simulink model "test_pi_av_formation_event_gazebodirected23a"  (R2023a)
settings: Solver=FixedStepAuto  StartTime=0.0  StopTime=inf  RelTol=1e-3
undefined symbols (not defined in the file or in its folder): angular, DiscIntNeverNeededParam, linear
libraries: ros2lib x28, simulink x8, robotcorelib x8
(part 3 of 4)

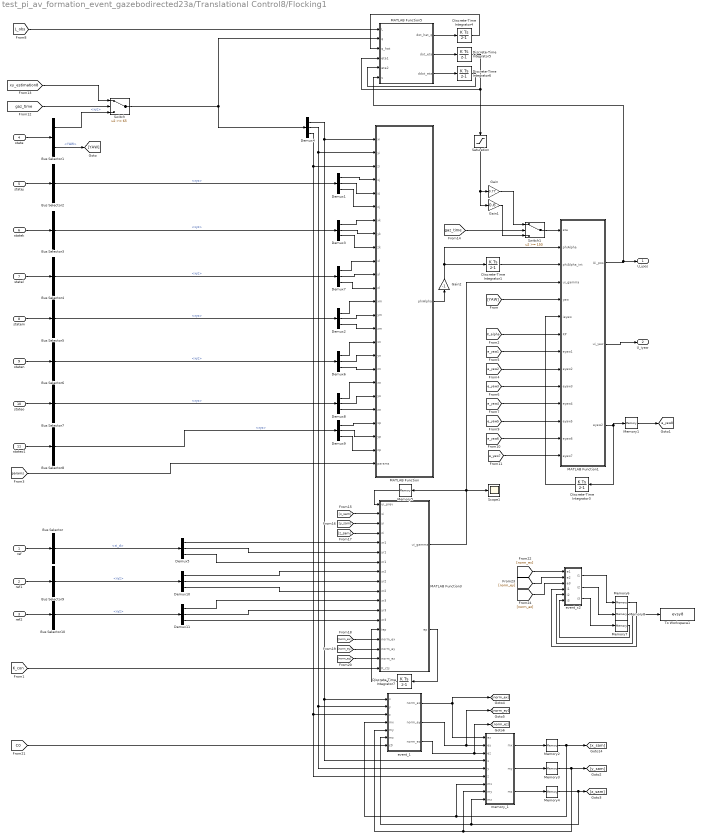
== system test_pi_av_formation_event_gazebodirected23a/Translational Control8/Flocking1 ==
  ref : Inport
  ref1 : Inport  Port=2
  ref2 : Inport  Port=3
  state : Inport  Port=4
  statej : Inport  Port=5
  statek : Inport  Port=6
  statel : Inport  Port=7
  statem : Inport  Port=8
  staten : Inport  Port=9
  stateo : Inport  Port=10
  stateo1 : Inport  Port=11
  Bus Selector : BusSelector  OutputSignals=xi_d
  Bus Selector1 : BusSelector  OutputSignals=xyz,YAW
  Bus Selector{2..10} (9 alike) : BusSelector  OutputSignals=xyz
  Demux{1..11} (11 alike) : Demux  Outputs=3
  Discrete-Time Integrator1 : DiscreteIntegrator  SampleTime=-1  LimitOutput=on  UpperSaturationLimit=2  LowerSaturationLimit=-2  ICPrevOutput=DiscIntNeverNeededParam  ICPrevScaledInput=DiscIntNeverNeededParam
  Discrete-Time Integrator3 : DiscreteIntegrator  SampleTime=-1  LimitOutput=on  UpperSaturationLimit=1  LowerSaturationLimit=-1  ICPrevOutput=DiscIntNeverNeededParam  ICPrevScaledInput=DiscIntNeverNeededParam
  Discrete-Time Integrator4 : DiscreteIntegrator  SampleTime=-1  LimitOutput=on  UpperSaturationLimit=5  LowerSaturationLimit=-5  ICPrevOutput=DiscIntNeverNeededParam  ICPrevScaledInput=DiscIntNeverNeededParam
  Discrete-Time Integrator5 : DiscreteIntegrator  SampleTime=-1  LimitOutput=on  UpperSaturationLimit=5  LowerSaturationLimit=-5  ICPrevOutput=DiscIntNeverNeededParam  ICPrevScaledInput=DiscIntNeverNeededParam
  Discrete-Time Integrator6 : DiscreteIntegrator  SampleTime=-1  LimitOutput=on  UpperSaturationLimit=0.4  LowerSaturationLimit=-0.4  ICPrevOutput=DiscIntNeverNeededParam  ICPrevScaledInput=DiscIntNeverNeededParam
  Discrete-Time Integrator7 : DiscreteIntegrator  SampleTime=-1  LimitOutput=on  UpperSaturationLimit=2  LowerSaturationLimit=-2  ICPrevOutput=DiscIntNeverNeededParam  ICPrevScaledInput=DiscIntNeverNeededParam
  Gain : Gain  Gain=0.77
  Gain1 : Gain  Gain=0.6
  Gain2 : Gain  Gain=-1
  MATLAB Function : MATLAB Function  TreatAsAtomicUnit=on
  MATLAB Function1 : MATLAB Function  TreatAsAtomicUnit=on
  MATLAB Function3 : MATLAB Function  TreatAsAtomicUnit=on
  MATLAB Function5 : MATLAB Function  TreatAsAtomicUnit=on
  Memory1 : Memory  InitialCondition=1
  Memory{2..4,6..8} (6 alike) : Memory
  Memory5 : Memory  InitialCondition=[0 0 0]'
  Saturation : Saturate  UpperLimit=1  LowerLimit=-1
  Scope1 : Scope
  Switch : Switch  Threshold=65  SaturateOnIntegerOverflow=off  InputSameDT=off
  Switch1 : Switch  Threshold=150  SaturateOnIntegerOverflow=off  InputSameDT=off
  To Workspace1 : ToWorkspace  VariableName=evsy8  SampleTime=-1
  event_1 : MATLAB Function  TreatAsAtomicUnit=on
  event_x2 : MATLAB Function  TreatAsAtomicUnit=on
  memory_1 : MATLAB Function  TreatAsAtomicUnit=on
  U_ipos : Outport  VectorParamsAs1DForOutWhenUnconnected=off
  U_iyaw : Outport  Port=2  VectorParamsAs1DForOutWhenUnconnected=off
  tag scope: e_yaw8=global
  wires:
  [e_yaw7] -> MATLAB Function1/14(eyaw7)
  Bus Selector8/1 -> Demux9/1  "<xyz>"
  Demux9/3 -> MATLAB Function/24(zp)
  Demux9/1 -> MATLAB Function/22(xp)
  Demux9/2 -> MATLAB Function/23(yp)
  stateo1/1 -> Bus Selector8/1
  ref/1 -> Bus Selector/1
  state/1 -> Bus Selector1/1
  Bus Selector/1 -> Demux5/1  "<xi_d>"
  statej/1 -> Bus Selector2/1
  Bus Selector2/1 -> Demux1/1  "<xyz>"
  Demux1/1 -> MATLAB Function/4(xj)
  Demux1/2 -> MATLAB Function/5(yj)
  Discrete-Time Integrator1/1 -> MATLAB Function1/3(phiAlpha_int)
  statek/1 -> Bus Selector3/1
  Demux3/1 -> MATLAB Function/7(xk)
  Demux3/2 -> MATLAB Function/8(yk)
  Bus Selector3/1 -> Demux3/1  "<xyz>"
  MATLAB Function/1(phiAlpha) -> Gain2/1
  Demux3/3 -> MATLAB Function/9(zk)
  Demux1/3 -> MATLAB Function/6(zj)
  statel/1 -> Bus Selector4/1
  Demux7/1 -> MATLAB Function/10(xl)
  Demux7/2 -> MATLAB Function/11(yl)
  Demux7/3 -> MATLAB Function/12(zl)
  Bus Selector4/1 -> Demux7/1  "<xyz>"
  Bus Selector1/2 -> [YAW]  "<YAW>"
  [YAW] -> MATLAB Function1/5(yaw)
  MATLAB Function1/2(ui_yaw) -> U_iyaw/1
  MATLAB Function1/3(eyaw2) -> Discrete-Time Integrator3/1, Memory1/1
  Discrete-Time Integrator3/1 -> MATLAB Function1/6(ieyaw)
  [K_alpha] -> MATLAB Function1/7(KP)
  [params] -> MATLAB Function/25(params)
  statem/1 -> Bus Selector5/1
  Bus Selector5/1 -> Demux2/1  "<xyz>"
  Demux2/1 -> MATLAB Function/13(xm)
  Demux2/2 -> MATLAB Function/14(ym)
  Demux2/3 -> MATLAB Function/15(zm)
  Memory1/1 -> [e_yaw8]
  [e_yaw1] -> MATLAB Function1/8(eyaw1)
  [e_yaw3] -> MATLAB Function1/10(eyaw3)
  [e_yaw4] -> MATLAB Function1/11(eyaw4)
  [e_yaw2] -> MATLAB Function1/9("eyaw2 ")
  Discrete-Time Integrator4/1 -> MATLAB Function5/3(q_hat)
  Discrete-Time Integrator5/1 -> Saturation/1, MATLAB Function5/4(eta1)
  [L_obs] -> MATLAB Function5/1(L)
  MATLAB Function5/1(dot_hat_q) -> Discrete-Time Integrator4/1
  MATLAB Function1/1(Ui_pos) -> MATLAB Function5/6(u), U_ipos/1
  MATLAB Function5/2(dot_eta) -> Discrete-Time Integrator5/1
  Discrete-Time Integrator6/1 -> MATLAB Function5/5(eta2)
  MATLAB Function5/3(ddot_eta) -> Discrete-Time Integrator6/1
  staten/1 -> Bus Selector6/1
  Demux6/1 -> MATLAB Function/16(xn)
  Demux6/2 -> MATLAB Function/17(yn)
  Demux6/3 -> MATLAB Function/18(zn)
  Bus Selector6/1 -> Demux6/1  "<xyz>"
  [e_yaw5] -> MATLAB Function1/12(eyaw5)
  stateo/1 -> Bus Selector7/1
  Demux8/1 -> MATLAB Function/19(xo)
  Demux8/2 -> MATLAB Function/20(yo)
  Demux8/3 -> MATLAB Function/21(zo)
  Bus Selector7/1 -> Demux8/1  "<xyz>"
  [e_yaw6] -> MATLAB Function1/13(eyaw6)
  [xy_estimation8] -> Switch/1
  [gaz_time] -> Switch/2
  Bus Selector1/1 -> Switch/3  "<xyz>"
  Switch/1 -> MATLAB Function5/2(q), Demux4/1
  Bus Selector9/1 -> Demux10/1  "<xyz>"
  ref1/1 -> Bus Selector9/1
  ref2/1 -> Bus Selector10/1
  Bus Selector10/1 -> Demux11/1  "<xyz>"
  Saturation/1 -> Gain1/1, Gain/1
  Switch1/1 -> MATLAB Function1/1(eta)
  Gain1/1 -> Switch1/3
  Gain/1 -> Switch1/1
  [gaz_time] -> Switch1/2
  event_1/3(norm_ez) -> [norm_ez], memory_1/3(ez)
  Memory2/1 -> memory_1/7("mx "), event_1/4(mx), [x_sam]
  [norm_ez] -> MATLAB Function3/17(norm_ez)
  MATLAB Function3/1(ui_gamma) -> MATLAB Function1/4(ui_gamma), Scope1/1, Memory5/1
  Memory5/1 -> MATLAB Function3/1(ui_prev)
  memory_1/1(mx) -> Memory2/1
  Memory3/1 -> [y_sam], memory_1/8("my "), event_1/5(my)
  event_1/1(norm_ex) -> [norm_ex], memory_1/1(ex)
  memory_1/3(mz) -> Memory4/1
  MATLAB Function3/2(ep) -> Discrete-Time Integrator7/1
  [norm_ey] -> MATLAB Function3/16(norm_ey)
  [norm_ex] -> MATLAB Function3/15(norm_ex)
  memory_1/2(my) -> Memory3/1
  [x_sam] -> MATLAB Function3/2(xi)
  Discrete-Time Integrator7/1 -> MATLAB Function3/14(iep)
  event_1/2(norm_ey) -> [norm_ey], memory_1/2(ey)
  [y_sam] -> MATLAB Function3/3(yi)
  [z_sam] -> MATLAB Function3/4(zi)
  Demux4/1 -> memory_1/4(x), event_1/1(x), MATLAB Function/1(xi)
  Memory4/1 -> memory_1/9("mz "), event_1/6(mz), [z_sam]
  Demux4/2 -> memory_1/5(y), event_1/2(y), MATLAB Function/2(yi)
  Demux4/3 -> memory_1/6(z), event_1/3(z), MATLAB Function/3(zi)
  Demux11/1 -> MATLAB Function3/11(xr3)
  Demux10/1 -> MATLAB Function3/8(xr2)
  Demux11/2 -> MATLAB Function3/12(yr3)
  Demux5/1 -> MATLAB Function3/5(xr1)
  Demux10/2 -> MATLAB Function3/9(yr2)
  Demux11/3 -> MATLAB Function3/13(zr3)
  Demux5/2 -> MATLAB Function3/6(yr1)
  Demux10/3 -> MATLAB Function3/10(zr2)
  Demux5/3 -> MATLAB Function3/7(zr1)
  [K_con] -> MATLAB Function3/18(K_cts)
  [C0] -> event_1/7(c0)
  Gain2/1 -> MATLAB Function1/2(phiAlpha), Discrete-Time Integrator1/1
  Memory7/1 -> event_x2/6("i3 ")
  [norm_ez] -> event_x2/3(e3)
  [norm_ex] -> event_x2/1(e1)
  event_x2/2(i2) -> Memory8/1
  Memory8/1 -> To Workspace1/1, event_x2/5("i2 ")
  event_x2/1(i1) -> Memory6/1
  Memory6/1 -> event_x2/4("i1 ")
  event_x2/3(i3) -> Memory7/1
  [norm_ey] -> event_x2/2(e2)

== matlab function test_pi_av_formation_event_gazebodirected23a/Translational Control3/Flocking1/event_1 ==
  data: x input; y input; z input; mx input; my input; mz input; norm_ex output; norm_ey output; c0 input; norm_ez output
function [norm_ex, norm_ey, norm_ez] = fcn(x, y, z, mx, my, mz, c0)

cx = c0(1); cy = c0(2); cz = c0(3); 

norm_ex = abs((mx-x)) - cx;
norm_ey = abs((my-y)) - cy;
norm_ez = abs((mz-z)) - cz;

== matlab function test_pi_av_formation_event_gazebodirected23a/Translational Control3/Flocking1/memory_1 ==
  data: ex input; ey input; mx output; ez input; x input; y input; z input; mx input; my input; mz input; my output; mz output
function [mx, my, mz] = fcn(ex, ey, ez, x, y, z, mx, my, mz)

if ex >= 0
    mx = x;    
else
    mx = mx;
end

if ey >= 0
    my = y;    
else
    my = my;
end

if ez >= 0
    mz = z;    
else
    mz = mz;
end

== matlab function test_pi_av_formation_event_gazebodirected23a/Translational Control4/Flocking1/event_1 ==
  data: x input; y input; z input; mx input; my input; mz input; norm_ex output; norm_ey output; c0 input; norm_ez output
function [norm_ex, norm_ey, norm_ez] = fcn(x, y, z, mx, my, mz, c0)

cx = c0(1); cy = c0(2); cz = c0(3); 

norm_ex = abs((mx-x)) - cx;
norm_ey = abs((my-y)) - cy;
norm_ez = abs((mz-z)) - cz;

== matlab function test_pi_av_formation_event_gazebodirected23a/Translational Control4/Flocking1/memory_1 ==
  data: ex input; ey input; mx output; ez input; x input; y input; z input; mx input; my input; mz input; my output; mz output
function [mx, my, mz] = fcn(ex, ey, ez, x, y, z, mx, my, mz)

if ex >= 0
    mx = x;    
else
    mx = mx;
end

if ey >= 0
    my = y;    
else
    my = my;
end

if ez >= 0
    mz = z;    
else
    mz = mz;
end

== matlab function test_pi_av_formation_event_gazebodirected23a/MATLAB Function1 ==
  data: sec input; gaz_time output; nanosec input
function gaz_time = fcn(sec, nanosec)

nanosec1 = double(nanosec)/1000000000; %*10^(-9);

sec1 = double(sec);

gaz_time = sec1 + nanosec1;

== matlab function test_pi_av_formation_event_gazebodirected23a/Translational Control5/Flocking1/event_1 ==
  data: x input; y input; z input; mx input; my input; mz input; norm_ex output; norm_ey output; c0 input; norm_ez output
function [norm_ex, norm_ey, norm_ez] = fcn(x, y, z, mx, my, mz, c0)

cx = c0(1); cy = c0(2); cz = c0(3); 

norm_ex = abs((mx-x)) - cx;
norm_ey = abs((my-y)) - cy;
norm_ez = abs((mz-z)) - cz;

== matlab function test_pi_av_formation_event_gazebodirected23a/Translational Control5/Flocking1/memory_1 ==
  data: ex input; ey input; mx output; ez input; x input; y input; z input; mx input; my input; mz input; my output; mz output
function [mx, my, mz] = fcn(ex, ey, ez, x, y, z, mx, my, mz)

if ex >= 0
    mx = x;    
else
    mx = mx;
end

if ey >= 0
    my = y;    
else
    my = my;
end

if ez >= 0
    mz = z;    
else
    mz = mz;
end

== matlab function test_pi_av_formation_event_gazebodirected23a/Translational Control6/Flocking1/event_1 ==
  data: x input; y input; z input; mx input; my input; mz input; norm_ex output; norm_ey output; c0 input; norm_ez output
function [norm_ex, norm_ey, norm_ez] = fcn(x, y, z, mx, my, mz, c0)

cx = c0(1); cy = c0(2); cz = c0(3); 

norm_ex = abs((mx-x)) - cx;
norm_ey = abs((my-y)) - cy;
norm_ez = abs((mz-z)) - cz;

== matlab function test_pi_av_formation_event_gazebodirected23a/Translational Control6/Flocking1/memory_1 ==
  data: ex input; ey input; mx output; ez input; x input; y input; z input; mx input; my input; mz input; my output; mz output
function [mx, my, mz] = fcn(ex, ey, ez, x, y, z, mx, my, mz)

if ex >= 0
    mx = x;    
else
    mx = mx;
end

if ey >= 0
    my = y;    
else
    my = my;
end

if ez >= 0
    mz = z;    
else
    mz = mz;
end

== matlab function test_pi_av_formation_event_gazebodirected23a/Subsystem/dist_AVT ==
  data: meas input; u_B input; dU output; dAVT output; avt_pars input
function [dU,dAVT]  = fcn(meas, u_B, avt_pars)

%Vector separation
d1 = meas(1);
d2 = meas(2);
d3 = meas(3);
d4 = meas(4);
d5 = meas(5);
d6 = meas(6);
d7 = meas(7);

avtpars = avt_pars(1:4);
inc = avtpars(1);
dec = avtpars(2);
min = avtpars(3);
max = avtpars(4);

%% memory variables
d_avt1 = u_B(1);
adjustment1 = u_B(2);
s_adjust1 = u_B(3);

d_avt2 = u_B(4);
adjustment2 = u_B(5);
s_adjust2 = u_B(6);

d_avt3 = u_B(7);
adjustment3 = u_B(8);
s_adjust3 = u_B(9);

d_avt4 = u_B(10);
adjustment4 = u_B(11);
s_adjust4 = u_B(12);

d_avt5 = u_B(13);
adjustment5 = u_B(14);
s_adjust5 = u_B(15);

d_avt6 = u_B(16);
adjustment6 = u_B(17);
s_adjust6 = u_B(18);

d_avt7 = u_B(19);
adjustment7 = u_B(20);
s_adjust7 = u_B(21);

%%
du1 = AVTfun(d_avt1, d1, adjustment1, s_adjust1, min, max, inc, dec);

du2 = AVTfun(d_avt2, d2, adjustment2, s_adjust2, min, max, inc, dec);

du3 = AVTfun(d_avt3, d3, adjustment3, s_adjust3, min, max, inc, dec);

du4 = AVTfun(d_avt4, d4, adjustment4, s_adjust4, min, max, inc, dec);

du5 = AVTfun(d_avt5, d5, adjustment5, s_adjust5, min, max, inc, dec);

du6 = AVTfun(d_avt6, d6, adjustment6, s_adjust6, min, max, inc, dec);

du7 = AVTfun(d_avt7, d7, adjustment7, s_adjust7, min, max, inc, dec);

dU = [du1;du2;du3;du4;du5;du6;du7];
dAVT = [du1(1);du2(1);du3(1);du4(1);du5(1);du6(1);du7(1)];

== matlab function test_pi_av_formation_event_gazebodirected23a/MATLAB Function ==
  data: data input; y output
function y = fcn(data)

DATA = data(1:20);
d1 = awgn(double(DATA(1)), 33, 'measured');
d2 = awgn(double(DATA(2)), 33, 'measured');
d3 = awgn(double(DATA(3)), 33, 'measured');
d4 = awgn(double(DATA(4)), 33, 'measured');
d5 = awgn(double(DATA(5)), 33, 'measured');
d6 = awgn(double(DATA(6)), 33, 'measured');
d7 = awgn(double(DATA(7)), 33, 'measured');
y = [d1;d2;d3;d4;d5;d6;d7];

== matlab function test_pi_av_formation_event_gazebodirected23a/Subsystem/MATLAB Function6 ==
  data: X1 input; X2 input; X3 input; X4 input; X5 input; X6 input; X7 input; d_meas input; xyz output
function xyz = fcn(X1, X2, X3, X4, X5, X6, X7, d_meas)

%% Extract data from vectors
states1 = X1(1:3);
x1 = states1(1);
y1 = states1(2);
z1 = states1(3);

states2 = X2(1:3);
x2 = states2(1);
y2 = states2(2);
z2 = states2(3);

states3 = X3(1:3);
x3 = states3(1);
y3 = states3(2);
z3 = states3(3);

states4 = X4(1:3);
x4 = states4(1);
y4 = states4(2);
z4 = states4(3);

states5 = X5(1:3);
x5 = states5(1);
y5 = states5(2);
z5 = states5(3);

states6 = X6(1:3);
x6 = states6(1);
y6 = states6(2);
z6 = states6(3);

states7 = X7(1:3);
x7 = states7(1);
y7 = states7(2);
z7 = states7(3);

r1 = d_meas(1);
r2 = d_meas(2);
r3 = d_meas(3);
r4 = d_meas(4);
r5 = d_meas(5);
r6 = d_meas(6);
r7 = d_meas(7);

xyz = multi_fun2(x1, y1, z1, r1, x2, y2, z2, r2, x3, y3, z3, r3, x4, y4, z4, r4, x5, y5, z5, r5, x6, y6, z6, r6, x7, y7, z7, r7);

== matlab function test_pi_av_formation_event_gazebodirected23a/Translational Control7/Flocking1/event_1 ==
  data: x input; y input; z input; mx input; my input; mz input; norm_ex output; norm_ey output; c0 input; norm_ez output
function [norm_ex, norm_ey, norm_ez] = fcn(x, y, z, mx, my, mz, c0)

cx = c0(1); cy = c0(2); cz = c0(3); 

norm_ex = abs((mx-x)) - cx;
norm_ey = abs((my-y)) - cy;
norm_ez = abs((mz-z)) - cz;

== matlab function test_pi_av_formation_event_gazebodirected23a/Translational Control7/Flocking1/memory_1 ==
  data: ex input; ey input; mx output; ez input; x input; y input; z input; mx input; my input; mz input; my output; mz output
function [mx, my, mz] = fcn(ex, ey, ez, x, y, z, mx, my, mz)

if ex >= 0
    mx = x;    
else
    mx = mx;
end

if ey >= 0
    my = y;    
else
    my = my;
end

if ez >= 0
    mz = z;    
else
    mz = mz;
end

== matlab function test_pi_av_formation_event_gazebodirected23a/Translational Control8/Flocking1/event_1 ==
  data: x input; y input; z input; mx input; my input; mz input; norm_ex output; norm_ey output; c0 input; norm_ez output
function [norm_ex, norm_ey, norm_ez] = fcn(x, y, z, mx, my, mz, c0)

cx = c0(1); cy = c0(2); cz = c0(3); 

norm_ex = abs((mx-x)) - cx;
norm_ey = abs((my-y)) - cy;
norm_ez = abs((mz-z)) - cz;

== matlab function test_pi_av_formation_event_gazebodirected23a/Translational Control8/Flocking1/memory_1 ==
  data: ex input; ey input; mx output; ez input; x input; y input; z input; mx input; my input; mz input; my output; mz output
function [mx, my, mz] = fcn(ex, ey, ez, x, y, z, mx, my, mz)

if ex >= 0
    mx = x;    
else
    mx = mx;
end

if ey >= 0
    my = y;    
else
    my = my;
end

if ez >= 0
    mz = z;    
else
    mz = mz;
end

== matlab function test_pi_av_formation_event_gazebodirected23a/Virtual_leader ==
  data: t input; xi_d output; dxi_d output; Xd input
function [xi_d, dxi_d]  = fcn(t, Xd)
%#codegen

f = 1/110;
radius=2;   %radius in meters

sel=1;      %inputs or parameters dont work! only local vars ...

if sel == 1
    if t < 90
       xd     =  0.5;
       xdotd  =  0;
           
       yd     = 0.5;
       ydotd  = 0;
           
       zd     = 1.3;  
       zdotd  = 0; 
           
       xi_d =[xd; yd; zd];
       dxi_d=[xdotd; ydotd; zdotd]; 
       
    elseif t < 120
        xd     =  0.4;
        xdotd  =  0;
            
        yd     = -0.4;
        ydotd  = 0;
            
        zd     = 2.5;  
        zdotd  = 0; 
            
        xi_d =[xd; yd; zd];
        dxi_d=[xdotd; ydotd; zdotd]; 
        
    elseif t < 220
       xd     = radius*sin(2*pi*f*t);
       xdotd  = radius*2*pi*f*cos(2*pi*f*t);
            
       yd     = radius*cos(2*pi*f*t);
       ydotd  = -radius*2*pi*f*sin(2*pi*f*t);
            
       zd     = 3;  %radius*cos(2*pi*f*t) + 5;
       zdotd  = 0;  %-radius*2*pi*f*sin(2*pi*f*t);
           
       xi_d =[xd; yd; zd];
       dxi_d=[xdotd; ydotd; zdotd];
    else
        xd     =  1;
        xdotd  =  0;
            
        yd     = 1;
        ydotd  = 0;
            
        zd     = 2;  
        zdotd  = 0; 
            
        xi_d =[xd; yd; zd];
        dxi_d=[xdotd; ydotd; zdotd];        
    end
end

 if(sel==2)
     xd     =  Xd(1);
     xdotd  =  0;
          
     yd     = Xd(2);
     ydotd  = 0;
          
     zd     = Xd(3);  
     zdotd  = 0; 
          
     xi_d =[xd; yd; zd];
     dxi_d=[xdotd; ydotd; zdotd]; 
     
 end

== matlab function test_pi_av_formation_event_gazebodirected23a/Translational Control2/Flocking1/event_x2 ==
  data: e1 input; e2 input; e3 input; i1 output; i1 input; i2 input; i3 input; i2 output; i3 output
function [i1, i2, i3]  = fcn(e1, e2, e3, i1, i2, i3)

if e1 >= 0
    e_1 = 1;
    i1 = i1+1;
else 
    e_1 = 0;
    i1 = i1;
end

if e2 >= 0
    e_2 = 1;
    i2 = i2 + 1;
else 
    e_2 = 0;
    i2 = i2;
end

if e3 >= 0
    e_3 = 1;
    i3 = i3 + 1;
else 
    e_3 = 0;
    i3 = i3;
end

== matlab function test_pi_av_formation_event_gazebodirected23a/Translational Control3/Flocking1/event_x2 ==
  data: e1 input; e2 input; e3 input; i1 output; i1 input; i2 input; i3 input; i2 output; i3 output
function [i1, i2, i3]  = fcn(e1, e2, e3, i1, i2, i3)

if e1 >= 0
    e_1 = 1;
    i1 = i1+1;
else 
    e_1 = 0;
    i1 = i1;
end

if e2 >= 0
    e_2 = 1;
    i2 = i2 + 1;
else 
    e_2 = 0;
    i2 = i2;
end

if e3 >= 0
    e_3 = 1;
    i3 = i3 + 1;
else 
    e_3 = 0;
    i3 = i3;
end

== matlab function test_pi_av_formation_event_gazebodirected23a/Translational Control4/Flocking1/event_x2 ==
  data: e1 input; e2 input; e3 input; i1 output; i1 input; i2 input; i3 input; i2 output; i3 output
function [i1, i2, i3]  = fcn(e1, e2, e3, i1, i2, i3)

if e1 >= 0
    e_1 = 1;
    i1 = i1+1;
else 
    e_1 = 0;
    i1 = i1;
end

if e2 >= 0
    e_2 = 1;
    i2 = i2 + 1;
else 
    e_2 = 0;
    i2 = i2;
end

if e3 >= 0
    e_3 = 1;
    i3 = i3 + 1;
else 
    e_3 = 0;
    i3 = i3;
end

== matlab function test_pi_av_formation_event_gazebodirected23a/Translational Control5/Flocking1/event_x2 ==
  data: e1 input; e2 input; e3 input; i1 output; i1 input; i2 input; i3 input; i2 output; i3 output
function [i1, i2, i3]  = fcn(e1, e2, e3, i1, i2, i3)

if e1 >= 0
    e_1 = 1;
    i1 = i1+1;
else 
    e_1 = 0;
    i1 = i1;
end

if e2 >= 0
    e_2 = 1;
    i2 = i2 + 1;
else 
    e_2 = 0;
    i2 = i2;
end

if e3 >= 0
    e_3 = 1;
    i3 = i3 + 1;
else 
    e_3 = 0;
    i3 = i3;
end

== matlab function test_pi_av_formation_event_gazebodirected23a/Translational Control6/Flocking1/event_x2 ==
  data: e1 input; e2 input; e3 input; i1 output; i1 input; i2 input; i3 input; i2 output; i3 output
function [i1, i2, i3]  = fcn(e1, e2, e3, i1, i2, i3)

if e1 >= 0
    e_1 = 1;
    i1 = i1+1;
else 
    e_1 = 0;
    i1 = i1;
end

if e2 >= 0
    e_2 = 1;
    i2 = i2 + 1;
else 
    e_2 = 0;
    i2 = i2;
end

if e3 >= 0
    e_3 = 1;
    i3 = i3 + 1;
else 
    e_3 = 0;
    i3 = i3;
end

== matlab function test_pi_av_formation_event_gazebodirected23a/Translational Control7/Flocking1/event_x2 ==
  data: e1 input; e2 input; e3 input; i1 output; i1 input; i2 input; i3 input; i2 output; i3 output
function [i1, i2, i3]  = fcn(e1, e2, e3, i1, i2, i3)

if e1 >= 0
    e_1 = 1;
    i1 = i1+1;
else 
    e_1 = 0;
    i1 = i1;
end

if e2 >= 0
    e_2 = 1;
    i2 = i2 + 1;
else 
    e_2 = 0;
    i2 = i2;
end

if e3 >= 0
    e_3 = 1;
    i3 = i3 + 1;
else 
    e_3 = 0;
    i3 = i3;
end

== matlab function test_pi_av_formation_event_gazebodirected23a/Translational Control2/Flocking1/MATLAB Function ==
  data: xi input; yi input; zi input; phiAlpha output; xj input; yj input; zj input; xk input; yk input; zk input; xl input; yl input; zl input; xm input; ym input; zm input; xn input; yn input; zn input; xo input; yo input; zo input; xp input; yp input; zp input; params input

function phiAlpha  = phiAlphaFcn(xi, yi, zi, xj, yj, zj, xk, yk, zk, xl, yl, zl, xm, ym, zm, xn, yn, zn, xo, yo, zo, xp, yp, zp, params)
    
    % Flocking parameters
    epsilon = params(1); a = params(2); b = params(3); c = params(4); d = params(5); h = params(6);

    e = abs(a - b) / sqrt(4*a*b) ;

    cAlpha = sigmaNormFun(c, epsilon) ;
    dAlpha = sigmaNormFun(d, epsilon) ;

    %%
    Pi = [xi;yi;zi] ;

    Pj = [xj;yj;zj] ;
    Pk = [xk;yk;zk] ;
    Pl = [xl;yl;zl] ;
    Pm = [xm;ym;zm] ;
    Pn = [xn;yn;zn] ;
    Po = [xo;yo;zo] ;
    Pp = [xp;yp;zp] ;

    %%
    sigmaNormj = sigmaNormFun(Pj - Pi, epsilon) ;
    nij = gradSigmaFun(Pj - Pi, epsilon) ;
    
    sigmaNormk = sigmaNormFun(Pk - Pi, epsilon) ;
    nik = gradSigmaFun(Pk - Pi, epsilon) ;

    sigmaNorml = sigmaNormFun(Pl - Pi, epsilon) ;
    nil = gradSigmaFun(Pl - Pi, epsilon) ;

    sigmaNormm = sigmaNormFun(Pm - Pi, epsilon) ;
    nim = gradSigmaFun(Pm - Pi, epsilon) ;

    sigmaNormn = sigmaNormFun(Pn - Pi, epsilon) ;
    nin = gradSigmaFun(Pn - Pi, epsilon) ;

    sigmaNormo = sigmaNormFun(Po - Pi, epsilon) ;
    nio = gradSigmaFun(Po - Pi, epsilon) ;

    sigmaNormp = sigmaNormFun(Pp - Pi, epsilon) ;
    nip = gradSigmaFun(Pp - Pi, epsilon) ;

    %%
    sigma1j = sigma1Fun(sigmaNormj - dAlpha + e) ;
    sigma1k = sigma1Fun(sigmaNormk - dAlpha + e) ;
    sigma1l = sigma1Fun(sigmaNorml - dAlpha + e) ;
    sigma1m = sigma1Fun(sigmaNormm - dAlpha + e) ;
    sigma1n = sigma1Fun(sigmaNormn - dAlpha + e) ;
    sigma1o = sigma1Fun(sigmaNormo - dAlpha + e) ;
    sigma1p = sigma1Fun(sigmaNormp - dAlpha + e) ;
            
    %% Position
    phiAlphaj = 0.5 * bumpFcn(sigmaNormj/cAlpha,h) * ((a+b)*sigma1j + (a-b)) ;
    phiAlphanij = phiAlphaj.* nij ;
    
    phiAlphak = 0.5 * bumpFcn(sigmaNormk/cAlpha,h) * ((a+b)*sigma1k + (a-b)) ;
    phiAlphanik = phiAlphak.* nik ;

    phiAlphal = 0.5 * bumpFcn(sigmaNorml/cAlpha,h) * ((a+b)*sigma1l + (a-b)) ;
    phiAlphanil = phiAlphal.* nil ;

    phiAlpham = 0.5 * bumpFcn(sigmaNormm/cAlpha,h) * ((a+b)*sigma1m + (a-b)) ;
    phiAlphanim = phiAlpham.* nim ;

    phiAlphan = 0.5 * bumpFcn(sigmaNormn/cAlpha,h) * ((a+b)*sigma1n + (a-b)) ;
    phiAlphanin = phiAlphan.* nin ;

    phiAlphao = 0.5 * bumpFcn(sigmaNormo/cAlpha,h) * ((a+b)*sigma1o + (a-b)) ;
    phiAlphanio = phiAlphao.* nio ;

    phiAlphap = 0.5 * bumpFcn(sigmaNormp/cAlpha,h) * ((a+b)*sigma1p + (a-b)) ;
    phiAlphanip = phiAlphap.* nip ;


    phiAlpha = phiAlphanij + phiAlphanik + phiAlphanil + phiAlphanim + phiAlphanin + phiAlphanio + phiAlphanip;

    
end

== matlab function test_pi_av_formation_event_gazebodirected23a/Translational Control8/Flocking1/event_x2 ==
  data: e1 input; e2 input; e3 input; i1 output; i1 input; i2 input; i3 input; i2 output; i3 output
function [i1, i2, i3]  = fcn(e1, e2, e3, i1, i2, i3)

if e1 >= 0
    e_1 = 1;
    i1 = i1+1;
else 
    e_1 = 0;
    i1 = i1;
end

if e2 >= 0
    e_2 = 1;
    i2 = i2 + 1;
else 
    e_2 = 0;
    i2 = i2;
end

if e3 >= 0
    e_3 = 1;
    i3 = i3 + 1;
else 
    e_3 = 0;
    i3 = i3;
end

== matlab function test_pi_av_formation_event_gazebodirected23a/continuous ==
  data: i output; t input; tp input; tp output; i input
function [i,tp] = fcn(t,tp,i)


%u = 0.1*cos(1.5*t) + 0.05*sin(t);         % x-component of vector field
%v = 0.1*sin(3*t) - 0.06*sin(0.5*t);      % y-component of vector field
if t > tp
    i = i + 1;
else 
    i = i;
end

== matlab function test_pi_av_formation_event_gazebodirected23a/Translational Control2/Flocking1/MATLAB Function1 ==
  data: eta input; phiAlpha input; phiAlpha_int input; ui_gamma input; yaw input; ieyaw input; Ui_pos output size=3; ui_yaw output; KP input; eyaw output size=1; eyaw1 input; eyaw3 input; eyaw4 input; eyaw5 input; eyaw6 input; eyaw7 input; eyaw8 input

function [Ui_pos, ui_yaw, eyaw]  = ctrlLaw(eta, phiAlpha, phiAlpha_int, ui_gamma, yaw, ieyaw, KP, eyaw1, eyaw3, eyaw4, eyaw5, eyaw6, eyaw7, eyaw8)  %, phiBetak, bikobs, phiBetanei, bikve
    
    % Control gains and parameters
    Kx = KP(1); Ky = KP(2); Kz = KP(3);
    Kix = KP(4); Kiy = KP(5); Kiz = KP(6);
    Kyaw = KP(7); Kdyaw = KP(8); Kiyaw = KP(9);
    offset = KP(10);

    eyaw = 0 - yaw(1);
    deyaw = 0 - yaw(2);

    ui_yaw = Kyaw*eyaw + Kdyaw*deyaw + Kiyaw*ieyaw;
    hz_dot = Kz * phiAlpha(3,1) + Kiz * phiAlpha_int(3,1) + ui_gamma(3,1) - eta(3,1);  
    
    if eyaw < offset && eyaw > -offset && eyaw1 < offset && eyaw1 > -offset && eyaw3 < offset && eyaw3 > -offset && eyaw4 < offset && eyaw4 > -offset && eyaw5 < offset && eyaw5 > -offset && eyaw6 < offset && eyaw6 > -offset && eyaw7 < offset && eyaw7 > -offset && eyaw8 < offset && eyaw8 > -offset
        hx_dot = Kx * phiAlpha(1,1) + Kix * phiAlpha_int(1,1) + ui_gamma(1,1) - eta(1,1);  
        hy_dot = Ky * phiAlpha(2,1) + Kiy * phiAlpha_int(2,1) + ui_gamma(2,1) - eta(2,1);  
    else
        hx_dot = 0;
        hy_dot = 0;
    end

    Ui_pos = [hx_dot; hy_dot; hz_dot] ;
    

end

== matlab function test_pi_av_formation_event_gazebodirected23a/Translational Control3/Flocking1/MATLAB Function3 ==
  data: ui_prev input; xi input; yi input; zi input; ui_gamma output; xr1 input; yr1 input; zr1 input; xr2 input; yr2 input; zr2 input; iep input size=3; norm_ex input; norm_ey input; norm_ez input; ep output size=3; K_cts input

function [ui_gamma, ep] = naviFeedback(ui_prev, xi, yi, zi, xr1, yr1, zr1, xr2, yr2, zr2, iep, norm_ex, norm_ey, norm_ez, K_cts)
    
    Kpxy = K_cts(1); Kixy = K_cts(2);
    xmin_xy = K_cts(3); xmax_xy = K_cts(4);
    Kpz = K_cts(5); Kiz = K_cts(6);
    xmin_z = K_cts(7); xmax_z = K_cts(8);

    %Sepration control
    ui_xprev = ui_prev(1); ui_yprev = ui_prev(2); ui_zprev = ui_prev(3);

%Errors
    e_x = (xi - xr1 - 0.55) + (xi - xr2);

    e_y = (yi - yr1 - 0.55) + (yi - yr2);

    e_z = (zi - zr1 + 0.55) + (zi - zr2 + 1.1);
       
    ep = [e_x;e_y;e_z];

    if  norm_ex >= 0
        ui_gammax = (-1)* satFcn_esc(Kpxy*e_x, xmin_xy, xmax_xy) + (-1)* satFcn_esc(Kixy*iep(1), xmin_xy, xmax_xy);
    else
        ui_gammax = ui_xprev;
    end

    if  norm_ey >= 0
        ui_gammay = (-1)* satFcn_esc(Kpxy*e_y, xmin_xy, xmax_xy) + (-1)* satFcn_esc(Kixy*iep(1), xmin_xy, xmax_xy);
    else
        ui_gammay = ui_yprev;
    end

    if  norm_ez >= 0
        ui_gammaz = (-1)* satFcn_esc(Kpz*e_z, xmin_z, xmax_z) + (-1)*satFcn_esc(Kiz*iep(3), xmin_z, xmax_z);
    else
        ui_gammaz = ui_zprev;
    end
    

    ui_gamma = [ui_gammax;ui_gammay;ui_gammaz];
    
end

== matlab function test_pi_av_formation_event_gazebodirected23a/Translational Control6/Flocking1/MATLAB Function ==
  data: xi input; yi input; zi input; phiAlpha output; xj input; yj input; zj input; xk input; yk input; zk input; xl input; yl input; zl input; xm input; ym input; zm input; xn input; yn input; zn input; xo input; yo input; zo input; xp input; yp input; zp input; params input

function phiAlpha  = phiAlphaFcn(xi, yi, zi, xj, yj, zj, xk, yk, zk, xl, yl, zl, xm, ym, zm, xn, yn, zn, xo, yo, zo, xp, yp, zp, params)
    
    % Flocking parameters
    epsilon = params(1); a = params(2); b = params(3); c = params(4); d = params(5); h = params(6);

    e = abs(a - b) / sqrt(4*a*b) ;

    cAlpha = sigmaNormFun(c, epsilon) ;
    dAlpha = sigmaNormFun(d, epsilon) ;

    %%
    Pi = [xi;yi;zi] ;

    Pj = [xj;yj;zj] ;
    Pk = [xk;yk;zk] ;
    Pl = [xl;yl;zl] ;
    Pm = [xm;ym;zm] ;
    Pn = [xn;yn;zn] ;
    Po = [xo;yo;zo] ;
    Pp = [xp;yp;zp] ;

    %%
    sigmaNormj = sigmaNormFun(Pj - Pi, epsilon) ;
    nij = gradSigmaFun(Pj - Pi, epsilon) ;
    
    sigmaNormk = sigmaNormFun(Pk - Pi, epsilon) ;
    nik = gradSigmaFun(Pk - Pi, epsilon) ;

    sigmaNorml = sigmaNormFun(Pl - Pi, epsilon) ;
    nil = gradSigmaFun(Pl - Pi, epsilon) ;

    sigmaNormm = sigmaNormFun(Pm - Pi, epsilon) ;
    nim = gradSigmaFun(Pm - Pi, epsilon) ;

    sigmaNormn = sigmaNormFun(Pn - Pi, epsilon) ;
    nin = gradSigmaFun(Pn - Pi, epsilon) ;

    sigmaNormo = sigmaNormFun(Po - Pi, epsilon) ;
    nio = gradSigmaFun(Po - Pi, epsilon) ;

    sigmaNormp = sigmaNormFun(Pp - Pi, epsilon) ;
    nip = gradSigmaFun(Pp - Pi, epsilon) ;

    %%
    sigma1j = sigma1Fun(sigmaNormj - dAlpha + e) ;
    sigma1k = sigma1Fun(sigmaNormk - dAlpha + e) ;
    sigma1l = sigma1Fun(sigmaNorml - dAlpha + e) ;
    sigma1m = sigma1Fun(sigmaNormm - dAlpha + e) ;
    sigma1n = sigma1Fun(sigmaNormn - dAlpha + e) ;
    sigma1o = sigma1Fun(sigmaNormo - dAlpha + e) ;
    sigma1p = sigma1Fun(sigmaNormp - dAlpha + e) ;
            
    %% Position
    phiAlphaj = 0.5 * bumpFcn(sigmaNormj/cAlpha,h) * ((a+b)*sigma1j + (a-b)) ;
    phiAlphanij = phiAlphaj.* nij ;
    
    phiAlphak = 0.5 * bumpFcn(sigmaNormk/cAlpha,h) * ((a+b)*sigma1k + (a-b)) ;
    phiAlphanik = phiAlphak.* nik ;

    phiAlphal = 0.5 * bumpFcn(sigmaNorml/cAlpha,h) * ((a+b)*sigma1l + (a-b)) ;
    phiAlphanil = phiAlphal.* nil ;

    phiAlpham = 0.5 * bumpFcn(sigmaNormm/cAlpha,h) * ((a+b)*sigma1m + (a-b)) ;
    phiAlphanim = phiAlpham.* nim ;

    phiAlphan = 0.5 * bumpFcn(sigmaNormn/cAlpha,h) * ((a+b)*sigma1n + (a-b)) ;
    phiAlphanin = phiAlphan.* nin ;

    phiAlphao = 0.5 * bumpFcn(sigmaNormo/cAlpha,h) * ((a+b)*sigma1o + (a-b)) ;
    phiAlphanio = phiAlphao.* nio ;

    phiAlphap = 0.5 * bumpFcn(sigmaNormp/cAlpha,h) * ((a+b)*sigma1p + (a-b)) ;
    phiAlphanip = phiAlphap.* nip ;


    phiAlpha = phiAlphanij + phiAlphanik + phiAlphanil + phiAlphanim  + phiAlphanin + phiAlphanio + phiAlphanip;

    
end

== matlab function test_pi_av_formation_event_gazebodirected23a/Translational Control6/Flocking1/MATLAB Function1 ==
  data: eta input; phiAlpha input; phiAlpha_int input; ui_gamma input; yaw input; ieyaw input; Ui_pos output size=3; ui_yaw output; KP input; eyaw2 output size=1; eyaw1 input; eyaw2 input; eyaw3 input; eyaw4 input; eyaw5 input; eyaw7 input; eyaw8 input

function [Ui_pos, ui_yaw, eyaw2]  = ctrlLaw(eta, phiAlpha, phiAlpha_int, ui_gamma, yaw, ieyaw, KP, eyaw1, eyaw2, eyaw3, eyaw4, eyaw5, eyaw7, eyaw8)  %, phiBetak, bikobs, phiBetanei, bikve
    
    % Control gains and parameters
    Kx = KP(1); Ky = KP(2); Kz = KP(3);
    Kix = KP(4); Kiy = KP(5); Kiz = KP(6);
    Kyaw = KP(7); Kdyaw = KP(8); Kiyaw = KP(9);
    offset = KP(10);

    eyaw = 0 - yaw(1);
    deyaw = 0 - yaw(2);

    ui_yaw = Kyaw*eyaw + Kdyaw*deyaw + Kiyaw*ieyaw;
    hz_dot = Kz * phiAlpha(3,1) + Kiz * phiAlpha_int(3,1) + ui_gamma(3,1) - eta(3,1);  
    
    if eyaw < offset && eyaw > -offset && eyaw1 < offset && eyaw1 > -offset && eyaw2 < offset && eyaw2 > -offset && eyaw3 < offset && eyaw3 > -offset && eyaw4 < offset && eyaw4 > -offset && eyaw5 < offset && eyaw5 > -offset && eyaw7 < offset && eyaw7 > -offset && eyaw8 < offset && eyaw8 > -offset
        hx_dot = Kx * phiAlpha(1,1) + Kix * phiAlpha_int(1,1) + ui_gamma(1,1) - eta(1,1);  
        hy_dot = Ky * phiAlpha(2,1) + Kiy * phiAlpha_int(2,1) + ui_gamma(2,1) - eta(2,1);  
    else
        hx_dot = 0;
        hy_dot = 0;
    end

    Ui_pos = [hx_dot; hy_dot; hz_dot] ;
    

end

== matlab function test_pi_av_formation_event_gazebodirected23a/Translational Control3/Flocking1/MATLAB Function ==
  data: xi input; yi input; zi input; phiAlpha output; xj input; yj input; zj input; xk input; yk input; zk input; xl input; yl input; zl input; xm input; ym input; zm input; xn input; yn input; zn input; xo input; yo input; zo input; xp input; yp input; zp input; params input

function phiAlpha  = phiAlphaFcn(xi, yi, zi, xj, yj, zj, xk, yk, zk, xl, yl, zl, xm, ym, zm, xn, yn, zn, xo, yo, zo, xp, yp, zp, params)
    
    % Flocking parameters
    epsilon = params(1); a = params(2); b = params(3); c = params(4); d = params(5); h = params(6);

    e = abs(a - b) / sqrt(4*a*b) ;

    cAlpha = sigmaNormFun(c, epsilon) ;
    dAlpha = sigmaNormFun(d, epsilon) ;

    %%
    Pi = [xi;yi;zi] ;

    Pj = [xj;yj;zj] ;
    Pk = [xk;yk;zk] ;
    Pl = [xl;yl;zl] ;
    Pm = [xm;ym;zm] ;
    Pn = [xn;yn;zn] ;
    Po = [xo;yo;zo] ;
    Pp = [xp;yp;zp] ;

    %%
    sigmaNormj = sigmaNormFun(Pj - Pi, epsilon) ;
    nij = gradSigmaFun(Pj - Pi, epsilon) ;
    
    sigmaNormk = sigmaNormFun(Pk - Pi, epsilon) ;
    nik = gradSigmaFun(Pk - Pi, epsilon) ;

    sigmaNorml = sigmaNormFun(Pl - Pi, epsilon) ;
    nil = gradSigmaFun(Pl - Pi, epsilon) ;

    sigmaNormm = sigmaNormFun(Pm - Pi, epsilon) ;
    nim = gradSigmaFun(Pm - Pi, epsilon) ;

    sigmaNormn = sigmaNormFun(Pn - Pi, epsilon) ;
    nin = gradSigmaFun(Pn - Pi, epsilon) ;

    sigmaNormo = sigmaNormFun(Po - Pi, epsilon) ;
    nio = gradSigmaFun(Po - Pi, epsilon) ;

    sigmaNormp = sigmaNormFun(Pp - Pi, epsilon) ;
    nip = gradSigmaFun(Pp - Pi, epsilon) ;

    %%
    sigma1j = sigma1Fun(sigmaNormj - dAlpha + e) ;
    sigma1k = sigma1Fun(sigmaNormk - dAlpha + e) ;
    sigma1l = sigma1Fun(sigmaNorml - dAlpha + e) ;
    sigma1m = sigma1Fun(sigmaNormm - dAlpha + e) ;
    sigma1n = sigma1Fun(sigmaNormn - dAlpha + e) ;
    sigma1o = sigma1Fun(sigmaNormo - dAlpha + e) ;
    sigma1p = sigma1Fun(sigmaNormp - dAlpha + e) ;
            
    %% Position
    phiAlphaj = 0.5 * bumpFcn(sigmaNormj/cAlpha,h) * ((a+b)*sigma1j + (a-b)) ;
    phiAlphanij = phiAlphaj.* nij ;
    
    phiAlphak = 0.5 * bumpFcn(sigmaNormk/cAlpha,h) * ((a+b)*sigma1k + (a-b)) ;
    phiAlphanik = phiAlphak.* nik ;

    phiAlphal = 0.5 * bumpFcn(sigmaNorml/cAlpha,h) * ((a+b)*sigma1l + (a-b)) ;
    phiAlphanil = phiAlphal.* nil ;

    phiAlpham = 0.5 * bumpFcn(sigmaNormm/cAlpha,h) * ((a+b)*sigma1m + (a-b)) ;
    phiAlphanim = phiAlpham.* nim ;

    phiAlphan = 0.5 * bumpFcn(sigmaNormn/cAlpha,h) * ((a+b)*sigma1n + (a-b)) ;
    phiAlphanin = phiAlphan.* nin ;

    phiAlphao = 0.5 * bumpFcn(sigmaNormo/cAlpha,h) * ((a+b)*sigma1o + (a-b)) ;
    phiAlphanio = phiAlphao.* nio ;


    phiAlpha = phiAlphanij + phiAlphanik + phiAlphanil + phiAlphanim + phiAlphanin + phiAlphanio;

    
end

== matlab function test_pi_av_formation_event_gazebodirected23a/Translational Control3/Flocking1/MATLAB Function1 ==
  data: eta input; phiAlpha input; phiAlpha_int input; ui_gamma input; yaw input; ieyaw input; Ui_pos output size=3; ui_yaw output; KP input; eyaw output size=1; eyaw1 input; eyaw2 input; eyaw4 input; eyaw5 input; eyaw6 input; eyaw7 input; eyaw8 input

function [Ui_pos, ui_yaw, eyaw]  = ctrlLaw(eta, phiAlpha, phiAlpha_int, ui_gamma, yaw, ieyaw, KP, eyaw1, eyaw2, eyaw4, eyaw5, eyaw6, eyaw7, eyaw8)  %, phiBetak, bikobs, phiBetanei, bikve
    
    % Control gains and parameters
    Kx = KP(1); Ky = KP(2); Kz = KP(3);
    Kix = KP(4); Kiy = KP(5); Kiz = KP(6);
    Kyaw = KP(7); Kdyaw = KP(8); Kiyaw = KP(9);
    offset = KP(10);

    eyaw = 0 - yaw(1);
    deyaw = 0 - yaw(2);

    ui_yaw = Kyaw*eyaw + Kdyaw*deyaw + Kiyaw*ieyaw;
    hz_dot = Kz * phiAlpha(3,1) + Kiz * phiAlpha_int(3,1) + ui_gamma(3,1) - eta(3,1);  
    
    if eyaw < offset && eyaw > -offset && eyaw1 < offset && eyaw1 > -offset && eyaw2 < offset && eyaw2 > -offset && eyaw4 < offset && eyaw4 > -offset && eyaw5 < offset && eyaw5 > -offset && eyaw6 < offset && eyaw6 > -offset && eyaw7 < offset && eyaw7 > -offset && eyaw8 < offset && eyaw8 > -offset
        hx_dot = Kx * phiAlpha(1,1) + Kix * phiAlpha_int(1,1) + ui_gamma(1,1) - eta(1,1);  
        hy_dot = Ky * phiAlpha(2,1) + Kiy * phiAlpha_int(2,1) + ui_gamma(2,1) - eta(2,1);  
    else
        hx_dot = 0;
        hy_dot = 0;
    end

    Ui_pos = [hx_dot; hy_dot; hz_dot] ;
    

end

== matlab function test_pi_av_formation_event_gazebodirected23a/Translational Control4/Flocking1/MATLAB Function3 ==
  data: ui_prev input; xi input; yi input; zi input; ui_gamma output; xr1 input; yr1 input; zr1 input; xr2 input; yr2 input; zr2 input; xr3 input; yr3 input; zr3 input; iep input size=3; norm_ex input; norm_ey input; norm_ez input; ep output size=3; K_cts input

function [ui_gamma, ep] = naviFeedback(ui_prev, xi, yi, zi, xr1, yr1, zr1, xr2, yr2, zr2, xr3, yr3, zr3, iep, norm_ex, norm_ey, norm_ez, K_cts)
    
    Kpxy = K_cts(1); Kixy = K_cts(2);
    xmin_xy = K_cts(3); xmax_xy = K_cts(4);
    Kpz = K_cts(5); Kiz = K_cts(6);
    xmin_z = K_cts(7); xmax_z = K_cts(8);

    %Sepration control
    ui_xprev = ui_prev(1); ui_yprev = ui_prev(2); ui_zprev = ui_prev(3);

%Errors
    e_x = (xi - xr1 + 0.55) + (xi - xr2 + 1.1)  + (xi - xr3 + 1.1);

    e_y = (yi - yr1 - 0.55) + (yi - yr2 - 1.1)  + (yi - yr3);

    e_z = (zi - zr1 + 0.55) + (zi - zr2)  + (zi - zr3 + 1.1);
       
    ep = [e_x;e_y;e_z];

    if  norm_ex >= 0
        ui_gammax = (-1)* satFcn_esc(Kpxy*e_x, xmin_xy, xmax_xy) + (-1)* satFcn_esc(Kixy*iep(1), xmin_xy, xmax_xy);
    else
        ui_gammax = ui_xprev;
    end

    if  norm_ey >= 0
        ui_gammay = (-1)* satFcn_esc(Kpxy*e_y, xmin_xy, xmax_xy) + (-1)* satFcn_esc(Kixy*iep(1), xmin_xy, xmax_xy);
    else
        ui_gammay = ui_yprev;
    end

    if  norm_ez >= 0
        ui_gammaz = (-1)* satFcn_esc(Kpz*e_z, xmin_z, xmax_z) + (-1)*satFcn_esc(Kiz*iep(3), xmin_z, xmax_z);
    else
        ui_gammaz = ui_zprev;
    end
    

    ui_gamma = [ui_gammax;ui_gammay;ui_gammaz];
    
end

== matlab function test_pi_av_formation_event_gazebodirected23a/Translational Control7/Flocking1/MATLAB Function3 ==
  data: ui_prev input; xi input; yi input; zi input; ui_gamma output; xr1 input; yr1 input; zr1 input; xr2 input; yr2 input; zr2 input; xr3 input; yr3 input; zr3 input; iep input size=3; norm_ex input; norm_ey input; norm_ez input; ep output size=3; K_cts input

function [ui_gamma, ep] = naviFeedback(ui_prev, xi, yi, zi, xr1, yr1, zr1, xr2, yr2, zr2, xr3, yr3, zr3, iep, norm_ex, norm_ey, norm_ez, K_cts)
    
    Kpxy = K_cts(1); Kixy = K_cts(2);
    xmin_xy = K_cts(3); xmax_xy = K_cts(4);
    Kpz = K_cts(5); Kiz = K_cts(6);
    xmin_z = K_cts(7); xmax_z = K_cts(8);

    %Sepration control
    ui_xprev = ui_prev(1); ui_yprev = ui_prev(2); ui_zprev = ui_prev(3);

%Errors
    e_x = (xi - xr1 - 0.55) + (xi - xr2)  + (xi - xr3);

    e_y = (yi - yr1 - 0.55) + (yi - yr2) + (yi - yr3 - 1.1);

    e_z = (zi - zr1 - 0.55) + (zi - zr2 - 1.1) + (zi - zr3 - 1.1);
       
    ep = [e_x;e_y;e_z];

    if  norm_ex >= 0
        ui_gammax = (-1)* satFcn_esc(Kpxy*e_x, xmin_xy, xmax_xy) + (-1)* satFcn_esc(Kixy*iep(1), xmin_xy, xmax_xy);
    else
        ui_gammax = ui_xprev;
    end

    if  norm_ey >= 0
        ui_gammay = (-1)* satFcn_esc(Kpxy*e_y, xmin_xy, xmax_xy) + (-1)* satFcn_esc(Kixy*iep(1), xmin_xy, xmax_xy);
    else
        ui_gammay = ui_yprev;
    end

    if  norm_ez >= 0
        ui_gammaz = (-1)* satFcn_esc(Kpz*e_z, xmin_z, xmax_z) + (-1)*satFcn_esc(Kiz*iep(3), xmin_z, xmax_z);
    else
        ui_gammaz = ui_zprev;
    end
    

    ui_gamma = [ui_gammax;ui_gammay;ui_gammaz];
    
end

== matlab function test_pi_av_formation_event_gazebodirected23a/Translational Control6/Flocking1/MATLAB Function5 ==
  data: dot_hat_q output; L input; q input; q_hat input; eta1 input; eta2 input; u input; dot_eta output; ddot_eta output
function [dot_hat_q, dot_eta, ddot_eta] = fcn(L, q, q_hat, eta1, eta2, u)

%%separation gains vectors
l2 = [L(1) L(2) L(3)];
l1 = [L(4) L(5) L(6)];
l0 = [L(7) L(8) L(9)];

L_2 = diag(l2);
L_1 = diag(l1);
L_0 = diag(l0);

dot_hat_q = q_est(u, eta1, L_2, q, q_hat);

dot_eta = dot_eta_one(eta2, L_1, q, q_hat);

ddot_eta = dot_eta_two(L_0, q, q_hat);

== matlab function test_pi_av_formation_event_gazebodirected23a/Translational Control4/Flocking1/MATLAB Function ==
  data: xi input; yi input; zi input; phiAlpha output; xj input; yj input; zj input; xk input; yk input; zk input; xl input; yl input; zl input; xm input; ym input; zm input; xn input; yn input; zn input; xo input; yo input; zo input; xp input; yp input; zp input; params input

function phiAlpha  = phiAlphaFcn(xi, yi, zi, xj, yj, zj, xk, yk, zk, xl, yl, zl, xm, ym, zm, xn, yn, zn, xo, yo, zo, xp, yp, zp, params)
    
    % Flocking parameters
    epsilon = params(1); a = params(2); b = params(3); c = params(4); d = params(5); h = params(6);

    e = abs(a - b) / sqrt(4*a*b) ;

    cAlpha = sigmaNormFun(c, epsilon) ;
    dAlpha = sigmaNormFun(d, epsilon) ;

    %%
    Pi = [xi;yi;zi] ;

    Pj = [xj;yj;zj] ;
    Pk = [xk;yk;zk] ;
    Pl = [xl;yl;zl] ;
    Pm = [xm;ym;zm] ;
    Pn = [xn;yn;zn] ;
    Po = [xo;yo;zo] ;
    Pp = [xp;yp;zp] ;

    %%
    sigmaNormj = sigmaNormFun(Pj - Pi, epsilon) ;
    nij = gradSigmaFun(Pj - Pi, epsilon) ;
    
    sigmaNormk = sigmaNormFun(Pk - Pi, epsilon) ;
    nik = gradSigmaFun(Pk - Pi, epsilon) ;

    sigmaNorml = sigmaNormFun(Pl - Pi, epsilon) ;
    nil = gradSigmaFun(Pl - Pi, epsilon) ;

    sigmaNormm = sigmaNormFun(Pm - Pi, epsilon) ;
    nim = gradSigmaFun(Pm - Pi, epsilon) ;

    sigmaNormn = sigmaNormFun(Pn - Pi, epsilon) ;
    nin = gradSigmaFun(Pn - Pi, epsilon) ;

    sigmaNormo = sigmaNormFun(Po - Pi, epsilon) ;
    nio = gradSigmaFun(Po - Pi, epsilon) ;

    sigmaNormp = sigmaNormFun(Pp - Pi, epsilon) ;
    nip = gradSigmaFun(Pp - Pi, epsilon) ;

    %%
    sigma1j = sigma1Fun(sigmaNormj - dAlpha + e) ;
    sigma1k = sigma1Fun(sigmaNormk - dAlpha + e) ;
    sigma1l = sigma1Fun(sigmaNorml - dAlpha + e) ;
    sigma1m = sigma1Fun(sigmaNormm - dAlpha + e) ;
    sigma1n = sigma1Fun(sigmaNormn - dAlpha + e) ;
    sigma1o = sigma1Fun(sigmaNormo - dAlpha + e) ;
    sigma1p = sigma1Fun(sigmaNormp - dAlpha + e) ;
            
    %% Position
    phiAlphaj = 0.5 * bumpFcn(sigmaNormj/cAlpha,h) * ((a+b)*sigma1j + (a-b)) ;
    phiAlphanij = phiAlphaj.* nij ;
    
    phiAlphak = 0.5 * bumpFcn(sigmaNormk/cAlpha,h) * ((a+b)*sigma1k + (a-b)) ;
    phiAlphanik = phiAlphak.* nik ;

    phiAlphal = 0.5 * bumpFcn(sigmaNorml/cAlpha,h) * ((a+b)*sigma1l + (a-b)) ;
    phiAlphanil = phiAlphal.* nil ;

    phiAlpham = 0.5 * bumpFcn(sigmaNormm/cAlpha,h) * ((a+b)*sigma1m + (a-b)) ;
    phiAlphanim = phiAlpham.* nim ;

    phiAlphan = 0.5 * bumpFcn(sigmaNormn/cAlpha,h) * ((a+b)*sigma1n + (a-b)) ;
    phiAlphanin = phiAlphan.* nin ;

    phiAlphao = 0.5 * bumpFcn(sigmaNormo/cAlpha,h) * ((a+b)*sigma1o + (a-b)) ;
    phiAlphanio = phiAlphao.* nio ;

    phiAlphap = 0.5 * bumpFcn(sigmaNormp/cAlpha,h) * ((a+b)*sigma1p + (a-b)) ;
    phiAlphanip = phiAlphap.* nip ;


    phiAlpha = phiAlphanij + phiAlphanik + phiAlphanil + phiAlphanim + phiAlphanin + phiAlphanio + phiAlphanip;

    
end

== matlab function test_pi_av_formation_event_gazebodirected23a/Translational Control4/Flocking1/MATLAB Function1 ==
  data: eta input; phiAlpha input; phiAlpha_int input; ui_gamma input; yaw input; ieyaw input; Ui_pos output size=3; ui_yaw output; KP input; eyaw output size=1; eyaw1 input; eyaw2 input; eyaw3 input; eyaw5 input; eyaw6 input; eyaw7 input; eyaw8 input
function [Ui_pos, ui_yaw, eyaw]  = ctrlLaw(eta, phiAlpha, phiAlpha_int, ui_gamma, yaw, ieyaw, KP, eyaw1, eyaw2, eyaw3, eyaw5, eyaw6, eyaw7, eyaw8)  %, phiBetak, bikobs, phiBetanei, bikve
    
    % Control gains and parameters
    Kx = KP(1); Ky = KP(2); Kz = KP(3);
    Kix = KP(4); Kiy = KP(5); Kiz = KP(6);
    Kyaw = KP(7); Kdyaw = KP(8); Kiyaw = KP(9);
    offset = KP(10);

    eyaw = 0 - yaw(1);
    deyaw = 0 - yaw(2);

    ui_yaw = Kyaw*eyaw + Kdyaw*deyaw + Kiyaw*ieyaw;
    hz_dot = Kz * phiAlpha(3,1) + Kiz * phiAlpha_int(3,1) + ui_gamma(3,1) - eta(3,1);  
    
    if eyaw < offset && eyaw > -offset && eyaw1 < offset && eyaw1 > -offset && eyaw2 < offset && eyaw2 > -offset && eyaw3 < offset && eyaw3 > -offset && eyaw5 < offset && eyaw5 > -offset && eyaw6 < offset && eyaw6 > -offset && eyaw7 < offset && eyaw7 > -offset && eyaw8 < offset && eyaw8 > -offset
        hx_dot = Kx * phiAlpha(1,1) + Kix * phiAlpha_int(1,1) + ui_gamma(1,1) - eta(1,1);  
        hy_dot = Ky * phiAlpha(2,1) + Kiy * phiAlpha_int(2,1) + ui_gamma(2,1) - eta(2,1);  
    else
        hx_dot = 0;
        hy_dot = 0;
    end

    Ui_pos = [hx_dot; hy_dot; hz_dot] ;
    

end

== matlab function test_pi_av_formation_event_gazebodirected23a/Translational Control1/Flocking1/MATLAB Function ==
  data: xi input; yi input; zi input; phiAlpha output; xj input; yj input; zj input; xk input; yk input; zk input; xl input; yl input; zl input; xm input; ym input; zm input; xn input; yn input; zn input; xo input; yo input; zo input; xp input; yp input; zp input; params input

function phiAlpha  = phiAlphaFcn(xi, yi, zi, xj, yj, zj, xk, yk, zk, xl, yl, zl, xm, ym, zm, xn, yn, zn, xo, yo, zo, xp, yp, zp, params)
    
    % Flocking parameters
    epsilon = params(1); a = params(2); b = params(3); c = params(4); d = params(5); h = params(6);

    e = abs(a - b) / sqrt(4*a*b) ;

    cAlpha = sigmaNormFun(c, epsilon) ;
    dAlpha = sigmaNormFun(d, epsilon) ;

    %%
    Pi = [xi;yi;zi] ;

    Pj = [xj;yj;zj] ;
    Pk = [xk;yk;zk] ;
    Pl = [xl;yl;zl] ;
    Pm = [xm;ym;zm] ;
    Pn = [xn;yn;zn] ;
    Po = [xo;yo;zo] ;
    Pp = [xp;yp;zp] ;

    %%
    sigmaNormj = sigmaNormFun(Pj - Pi, epsilon) ;
    nij = gradSigmaFun(Pj - Pi, epsilon) ;
    
    sigmaNormk = sigmaNormFun(Pk - Pi, epsilon) ;
    nik = gradSigmaFun(Pk - Pi, epsilon) ;

    sigmaNorml = sigmaNormFun(Pl - Pi, epsilon) ;
    nil = gradSigmaFun(Pl - Pi, epsilon) ;

    sigmaNormm = sigmaNormFun(Pm - Pi, epsilon) ;
    nim = gradSigmaFun(Pm - Pi, epsilon) ;

    sigmaNormn = sigmaNormFun(Pn - Pi, epsilon) ;
    nin = gradSigmaFun(Pn - Pi, epsilon) ;

    sigmaNormo = sigmaNormFun(Po - Pi, epsilon) ;
    nio = gradSigmaFun(Po - Pi, epsilon) ;

    sigmaNormp = sigmaNormFun(Pp - Pi, epsilon) ;
    nip = gradSigmaFun(Pp - Pi, epsilon) ;

    %%
    sigma1j = sigma1Fun(sigmaNormj - dAlpha + e) ;
    sigma1k = sigma1Fun(sigmaNormk - dAlpha + e) ;
    sigma1l = sigma1Fun(sigmaNorml - dAlpha + e) ;
    sigma1m = sigma1Fun(sigmaNormm - dAlpha + e) ;
    sigma1n = sigma1Fun(sigmaNormn - dAlpha + e) ;
    sigma1o = sigma1Fun(sigmaNormo - dAlpha + e) ;
    sigma1p = sigma1Fun(sigmaNormp - dAlpha + e) ;
            
    %% Position
    phiAlphaj = 0.5 * bumpFcn(sigmaNormj/cAlpha,h) * ((a+b)*sigma1j + (a-b)) ;
    phiAlphanij = phiAlphaj.* nij ;
    
    phiAlphak = 0.5 * bumpFcn(sigmaNormk/cAlpha,h) * ((a+b)*sigma1k + (a-b)) ;
    phiAlphanik = phiAlphak.* nik ;

    phiAlphal = 0.5 * bumpFcn(sigmaNorml/cAlpha,h) * ((a+b)*sigma1l + (a-b)) ;
    phiAlphanil = phiAlphal.* nil ;

    phiAlpham = 0.5 * bumpFcn(sigmaNormm/cAlpha,h) * ((a+b)*sigma1m + (a-b)) ;
    phiAlphanim = phiAlpham.* nim ;

    phiAlphan = 0.5 * bumpFcn(sigmaNormn/cAlpha,h) * ((a+b)*sigma1n + (a-b)) ;
    phiAlphanin = phiAlphan.* nin ;

    phiAlphao = 0.5 * bumpFcn(sigmaNormo/cAlpha,h) * ((a+b)*sigma1o + (a-b)) ;
    phiAlphanio = phiAlphao.* nio ;

    phiAlphap = 0.5 * bumpFcn(sigmaNormp/cAlpha,h) * ((a+b)*sigma1p + (a-b)) ;
    phiAlphanip = phiAlphap.* nip ;


    phiAlpha = phiAlphanij + phiAlphanik + phiAlphanil + phiAlphanim + phiAlphanin + phiAlphanio + phiAlphanip;

    
end

== matlab function test_pi_av_formation_event_gazebodirected23a/Translational Control1/Flocking1/MATLAB Function1 ==
  data: eta input; phiAlpha input; phiAlpha_int input; ui_gamma input; yaw input; ieyaw input; Ui_pos output size=3; ui_yaw output; KP input; eyaw output size=1; eyaw2 input; eyaw3 input; eyaw4 input; eyaw5 input; eyaw6 input; eyaw7 input; eyaw8 input

function [Ui_pos, ui_yaw, eyaw]  = ctrlLaw(eta, phiAlpha, phiAlpha_int, ui_gamma, yaw, ieyaw, KP, eyaw2, eyaw3, eyaw4, eyaw5, eyaw6, eyaw7, eyaw8)  %, phiBetak, bikobs, phiBetanei, bikve
    
    % Control gains and parameters
    Kx = KP(1); Ky = KP(2); Kz = KP(3);
    Kix = KP(4); Kiy = KP(5); Kiz = KP(6);
    Kyaw = KP(7); Kdyaw = KP(8); Kiyaw = KP(9);
    offset = KP(10);

    eyaw = 0 - yaw(1);
    deyaw = 0 - yaw(2);

    ui_yaw = Kyaw*eyaw + Kdyaw*deyaw + Kiyaw*ieyaw;
    hz_dot = Kz * phiAlpha(3,1) + Kiz * phiAlpha_int(3,1) + ui_gamma(3,1) - eta(3,1);  
    
    if eyaw < offset && eyaw > -offset && eyaw2 < offset && eyaw2 > -offset && eyaw3 < offset && eyaw3 > -offset && eyaw4 < offset && eyaw4 > -offset && eyaw5 < offset && eyaw5 > -offset && eyaw6 < offset && eyaw6 > -offset && eyaw7 < offset && eyaw7 > -offset && eyaw8 < offset && eyaw8 > -offset
        hx_dot = Kx * phiAlpha(1,1) + Kix * phiAlpha_int(1,1) + ui_gamma(1,1) - eta(1,1);  
        hy_dot = Ky * phiAlpha(2,1) + Kiy * phiAlpha_int(2,1) + ui_gamma(2,1) - eta(2,1);  
    else
        hx_dot = 0;
        hy_dot = 0;
    end

    Ui_pos = [hx_dot; hy_dot; hz_dot] ;
    

end
